simulink model "W02_3_goto_turtlesim"  (R2024b)
settings: Solver=FixedStepDiscrete  StartTime=0.0  StopTime=T_end  FixedStep=Ts  RelTol=1e-3
values from neighbouring files (symbols this model uses):
  animate = 1    [W02_setup.m]
  Kpsi = 4.0    (= 4)    [W02_setup.m]
  Kv = 1.0    (= 1)    [W02_setup.m]
  theta_goal = deg2rad(145)    [W02_setup.m]
  tol_d = 0.05    [W02_setup.m]
  tol_th = deg2rad(1.0)    [W02_setup.m]
  Ts = 0.05    [W02_setup.m]
  v_max = 2.0    (= 2)    [W02_setup.m]
  w_max = 2.0    (= 2)    [W02_setup.m]
  x_goal = 5.0    (= 5)    [W02_setup.m]
  y_goal = 5.0    (= 5)    [W02_setup.m]
undefined symbols (not defined in the file or in its folder): angular, linear
libraries: ros2lib x3
settings Model: Creator=admin  LastModifiedBy=admin

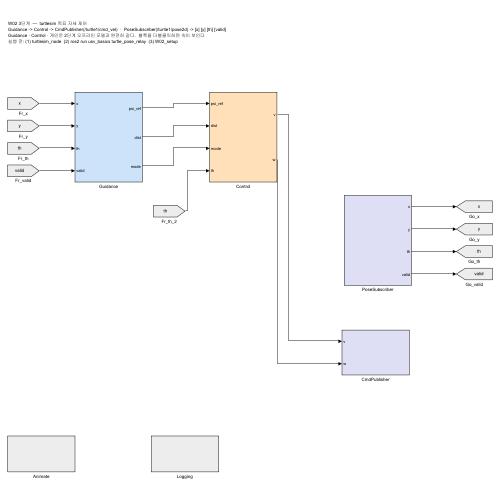
[thumbnail: Simulink's stored preview of the top-level diagram]
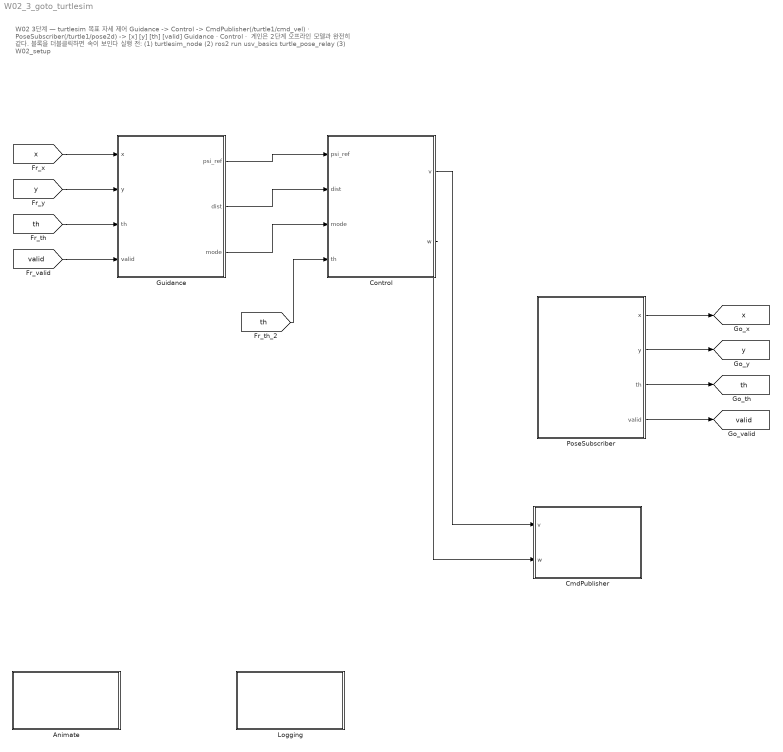
== system W02_3_goto_turtlesim ==
  note: W02 3단계  —  turtlesim 목표 자세 제어
      | Guidance -> Control -> CmdPublisher(/turtle1/cmd_vel)  ·  PoseSubscriber(/turtle1/pose2d) -> [x] [y] [th] [valid]
      | Guidance · Control · 게인은 2단계 오프라인 모델과 완전히 같다.  블록을 더블클릭하면 속이 보인다
      | 실행 전: (1) turtlesim_node  (2) ros2 run usv_basics turtle_pose_relay  (3) W02_setup
  Animate : Subsystem
  CmdPublisher : Subsystem
  Control : Subsystem
  Guidance : Subsystem
  Logging : Subsystem
  PoseSubscriber : Subsystem
  tag scope: th=global, valid=global, x=global, y=global
  wires:
  [x] -> Guidance/1(x)
  [y] -> Guidance/2(y)
  [th] -> Guidance/3(th)
  [valid] -> Guidance/4(valid)
  Guidance/1(psi_ref) -> Control/1(psi_ref)
  Guidance/2(dist) -> Control/2(dist)
  Guidance/3(mode) -> Control/3(mode)
  PoseSubscriber/1(x) -> [x]
  PoseSubscriber/2(y) -> [y]
  PoseSubscriber/3(th) -> [th]
  PoseSubscriber/4(valid) -> [valid]
  Control/2(w) -> CmdPublisher/2(w)
  Control/1(v) -> CmdPublisher/1(v)
  [th] -> Control/4(th)

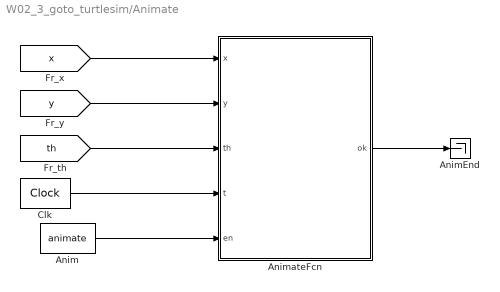
== system W02_3_goto_turtlesim/Animate ==
  Anim : Constant  Value=animate
  AnimEnd : Terminator
  AnimateFcn : MATLAB Function  TreatAsAtomicUnit=on
  Clk : DigitalClock  SampleTime=Ts
  wires:
  [x] -> AnimateFcn/1(x)
  [y] -> AnimateFcn/2(y)
  [th] -> AnimateFcn/3(th)
  Clk/1 -> AnimateFcn/4(t)
  Anim/1 -> AnimateFcn/5(en)
  AnimateFcn/1(ok) -> AnimEnd/1

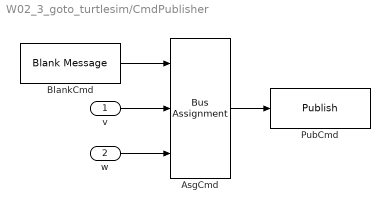
== system W02_3_goto_turtlesim/CmdPublisher ==
  v : Inport
  w : Inport  Port=2
  AsgCmd : BusAssignment  AssignedSignals=linear.x,angular.z
  BlankCmd : ros2lib/Blank Message  messageClass=Message  entityType=geometry_msgs/Twist  messageType=geometry_msgs/Twist  SampleTime=Ts
  PubCmd : ros2lib/Publish  topicSource=Specify your own  topic=/turtle1/cmd_vel  messageType=geometry_msgs/Twist  QOSHistory=Keep last  QOSDepth=1  QOSReliability=Reliable  QOSDurability=Volatile  QOSDeadline=Inf  QOSLifespan=Inf  QOSLiveliness=Automatic  QOSLeaseDuration=Inf  QOSAvoidROSNamespaceConventions=off
  wires:
  w/1 -> AsgCmd/3
  BlankCmd/1 -> AsgCmd/1
  v/1 -> AsgCmd/2
  AsgCmd/1 -> PubCmd/1

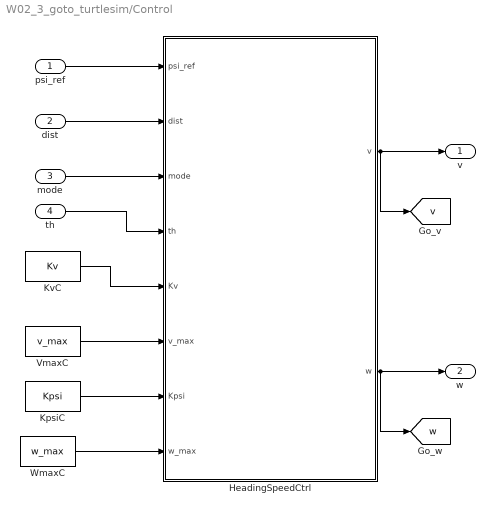
== system W02_3_goto_turtlesim/Control ==
  psi_ref : Inport
  dist : Inport  Port=2
  mode : Inport  Port=3
  th : Inport  Port=4
  HeadingSpeedCtrl : MATLAB Function  TreatAsAtomicUnit=on
  KpsiC : Constant  Value=Kpsi
  KvC : Constant  Value=Kv
  VmaxC : Constant  Value=v_max
  WmaxC : Constant  Value=w_max
  v : Outport
  w : Outport  Port=2
  tag scope: v=global, w=global
  wires:
  psi_ref/1 -> HeadingSpeedCtrl/1(psi_ref)
  dist/1 -> HeadingSpeedCtrl/2(dist)
  mode/1 -> HeadingSpeedCtrl/3(mode)
  KpsiC/1 -> HeadingSpeedCtrl/7(Kpsi)
  VmaxC/1 -> HeadingSpeedCtrl/6(v_max)
  th/1 -> HeadingSpeedCtrl/4(th)
  KvC/1 -> HeadingSpeedCtrl/5(Kv)
  WmaxC/1 -> HeadingSpeedCtrl/8(w_max)
  HeadingSpeedCtrl/1(v) -> v/1, [v]
  HeadingSpeedCtrl/2(w) -> w/1, [w]

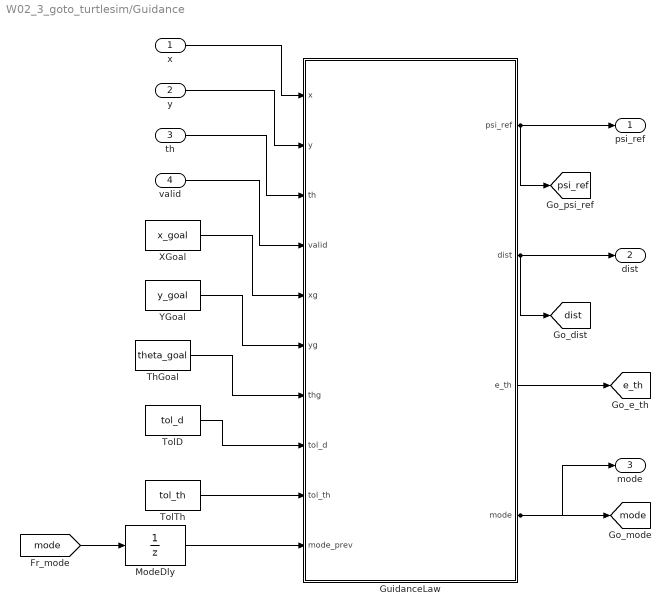
== system W02_3_goto_turtlesim/Guidance ==
  x : Inport
  y : Inport  Port=2
  th : Inport  Port=3
  valid : Inport  Port=4
  GuidanceLaw : MATLAB Function  TreatAsAtomicUnit=on
  ModeDly : UnitDelay  InitialCondition=1  SampleTime=Ts  HasFrameUpgradeWarning=on
  ThGoal : Constant  Value=theta_goal
  TolD : Constant  Value=tol_d
  TolTh : Constant  Value=tol_th
  XGoal : Constant  Value=x_goal
  YGoal : Constant  Value=y_goal
  psi_ref : Outport
  dist : Outport  Port=2
  mode : Outport  Port=3
  tag scope: dist=global, e_th=global, mode=global, psi_ref=global
  wires:
  XGoal/1 -> GuidanceLaw/5(xg)
  TolD/1 -> GuidanceLaw/8(tol_d)
  x/1 -> GuidanceLaw/1(x)
  YGoal/1 -> GuidanceLaw/6(yg)
  y/1 -> GuidanceLaw/2(y)
  th/1 -> GuidanceLaw/3(th)
  valid/1 -> GuidanceLaw/4(valid)
  ThGoal/1 -> GuidanceLaw/7(thg)
  TolTh/1 -> GuidanceLaw/9(tol_th)
  ModeDly/1 -> GuidanceLaw/10(mode_prev)
  GuidanceLaw/1(psi_ref) -> psi_ref/1, [psi_ref]
  GuidanceLaw/2(dist) -> dist/1, [dist]
  GuidanceLaw/3(e_th) -> [e_th]
  GuidanceLaw/4(mode) -> [mode], mode/1
  [mode] -> ModeDly/1

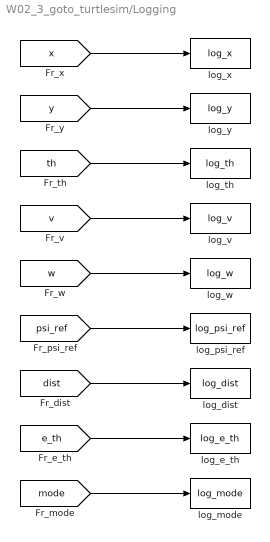
== system W02_3_goto_turtlesim/Logging ==
  log_dist : ToWorkspace  VariableName=log_dist  SaveFormat=Timeseries  SampleTime=Ts
  log_e_th : ToWorkspace  VariableName=log_e_th  SaveFormat=Timeseries  SampleTime=Ts
  log_mode : ToWorkspace  VariableName=log_mode  SaveFormat=Timeseries  SampleTime=Ts
  log_psi_ref : ToWorkspace  VariableName=log_psi_ref  SaveFormat=Timeseries  SampleTime=Ts
  log_th : ToWorkspace  VariableName=log_th  SaveFormat=Timeseries  SampleTime=Ts
  log_v : ToWorkspace  VariableName=log_v  SaveFormat=Timeseries  SampleTime=Ts
  log_w : ToWorkspace  VariableName=log_w  SaveFormat=Timeseries  SampleTime=Ts
  log_x : ToWorkspace  VariableName=log_x  SaveFormat=Timeseries  SampleTime=Ts
  log_y : ToWorkspace  VariableName=log_y  SaveFormat=Timeseries  SampleTime=Ts
  wires:
  [x] -> log_x/1
  [y] -> log_y/1
  [th] -> log_th/1
  [v] -> log_v/1
  [w] -> log_w/1
  [psi_ref] -> log_psi_ref/1
  [dist] -> log_dist/1
  [e_th] -> log_e_th/1
  [mode] -> log_mode/1

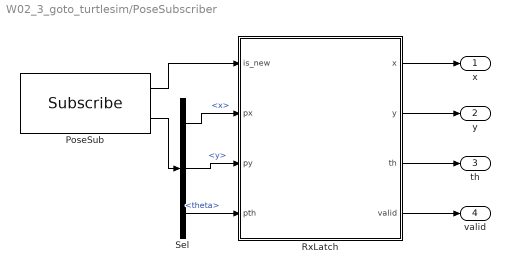
== system W02_3_goto_turtlesim/PoseSubscriber ==
  PoseSub : ros2lib/Subscribe  topicSource=Specify your own  topic=/turtle1/pose2d  messageType=geometry_msgs/Pose2D  sampleTime=Ts  QOSHistory=Keep last  QOSDepth=1  QOSReliability=Reliable  QOSDurability=Volatile  QOSDeadline=Inf  QOSLifespan=Inf  QOSLiveliness=Automatic  QOSLeaseDuration=Inf  QOSAvoidROSNamespaceConventions=off
  RxLatch : MATLAB Function  TreatAsAtomicUnit=on
  Sel : BusSelector  OutputSignals=x,y,theta
  x : Outport
  y : Outport  Port=2
  th : Outport  Port=3
  valid : Outport  Port=4
  wires:
  RxLatch/2(y) -> y/1
  Sel/2 -> RxLatch/3(py)  "<y>"
  PoseSub/1 -> RxLatch/1(is_new)
  PoseSub/2 -> Sel/1
  Sel/3 -> RxLatch/4(pth)  "<theta>"
  Sel/1 -> RxLatch/2(px)  "<x>"
  RxLatch/1(x) -> x/1
  RxLatch/3(th) -> th/1
  RxLatch/4(valid) -> valid/1

== matlab function W02_3_goto_turtlesim/Control/HeadingSpeedCtrl ==
  data: psi_ref input; v output; dist input; mode input; th input; Kv input; v_max input; Kpsi input; w_max input; w output
function [v, w] = HeadingSpeedCtrl(psi_ref, dist, mode, th, Kv, v_max, Kpsi, w_max)
%#codegen
% Heading control (P) and speed control (P on distance).
% turtlesim is kinematic: cmd_vel sets the velocity directly,
% so no yaw-rate (D) term or thrust model is needed here.

e = mod(psi_ref - th + pi, 2*pi) - pi;     % heading error, [-pi, pi)
w = min(max(Kpsi*e, -w_max), w_max);

if mode == 1
    % slow down near the goal; do not drive while facing away from it
    v = min(Kv*dist, v_max) * max(cos(e), 0);
elseif mode == 2
    v = 0;                                  % turn on the spot
else
    v = 0;  w = 0;                          % done
end

== matlab function W02_3_goto_turtlesim/Guidance/GuidanceLaw ==
  data: x input; psi_ref output; y input; th input; valid input; xg input; yg input; thg input; tol_d input; tol_th input; mode_prev input; dist output; e_th output; mode output
function [psi_ref, dist, e_th, mode] = GuidanceLaw(x, y, th, valid, xg, yg, thg, tol_d, tol_th, mode_prev)
%#codegen
% Go-to-pose guidance for turtlesim. One thing at a time:
%   mode 1 GO    : head for the goal point.   dist < tol_d   -> mode 2
%   mode 2 ALIGN : turn to the goal heading.  |e_th| < tol_th -> mode 3
%   mode 3 DONE  : stay still.  goal moved away (dist > 3*tol_d) -> mode 1
% turtlesim frame: x right, y up, theta counter-clockwise from +x.

dist = sqrt((xg - x)^2 + (yg - y)^2);
mode = mode_prev;

if valid < 0.5              % no pose received yet -> do not move
    psi_ref = th; e_th = 0; mode = 1;
    return
end

if mode == 1
    if dist < tol_d, mode = 2; end
elseif mode == 2
    if dist > 3*tol_d
        mode = 1;
    elseif abs(ssa(thg - th)) < tol_th
        mode = 3;
    end
else
    if dist > 3*tol_d, mode = 1; end
end

if mode == 1
    psi_ref = atan2(yg - y, xg - x);   % bearing to the goal point
else
    psi_ref = thg;                     % final heading
end
e_th = ssa(thg - th);                  % final-heading error (for logging)
end

function a = ssa(a)
% smallest signed angle, [-pi, pi)
a = mod(a + pi, 2*pi) - pi;
end

== matlab function W02_3_goto_turtlesim/PoseSubscriber/RxLatch ==
  data: x output; is_new input; y output; px input; py input; pth input; th output; valid output
function [x, y, th, valid] = RxLatch(is_new, px, py, pth)
%#codegen
% Before the first message arrives, Subscribe outputs an all-zero bus.
% (0,0) is a real corner of the turtlesim window, so it cannot be told
% apart by value. Latch the IsNew flag instead: valid = 0 until the
% first message, and Guidance keeps the turtle still until then.
persistent seen
if isempty(seen), seen = false; end
if is_new, seen = true; end
x = px;  y = py;  th = pth;
valid = double(seen);

== matlab function W02_3_goto_turtlesim/Animate/AnimateFcn ==
  data: x input; ok output; y input; th input; t input; en input
function ok = AnimateFcn(x, y, th, t, en)
%#codegen
% Live plot of the hull. Plotting is plain MATLAB, so it is
% declared extrinsic.
coder.extrinsic('W02_animate');
ok = 1;
if en > 0.5
    W02_animate(x, y, th, t);
end
